simulink model "auvDyn"  (R2018b)
settings: Solver=VariableStepAuto  StartTime=0.0  StopTime=3600  RelTol=1e-3
values from neighbouring files (symbols this model uses):
  aRef = auv.aRef.Value    [auvDyn_ts.m]    (also in hueristicAuvDyn_ts.m)
  AUVmass = auv.AUVmass.Value    [auvDyn_ts.m]    (also in hueristicAuvDyn_ts.m)
  cD = auv.cD.Value    [auvDyn_ts.m]    (also in hueristicAuvDyn_ts.m)
  floorFlow = .5    (= 0.5)    [auvDyn_ts.m]    (also in hueristicAuvDyn_ts.m)
  posOffset = auv.posOffset.Value    [auvDyn_ts.m]    (also in hueristicAuvDyn_ts.m)
  posSP = auv.posSP.Value    [auvDyn_ts.m]    (also in hueristicAuvDyn_ts.m)
  rho = auv.rho.Value    [auvDyn_ts.m]    (also in hueristicAuvDyn_ts.m)
libraries: filteredPIDController_ul x4, vrlib x1, sharedutil x1
settings Model: Creator=jcreed2  LastModifiedBy=jcreed2
settings DataIOCC: SaveOutput=off  DSMLogging=off

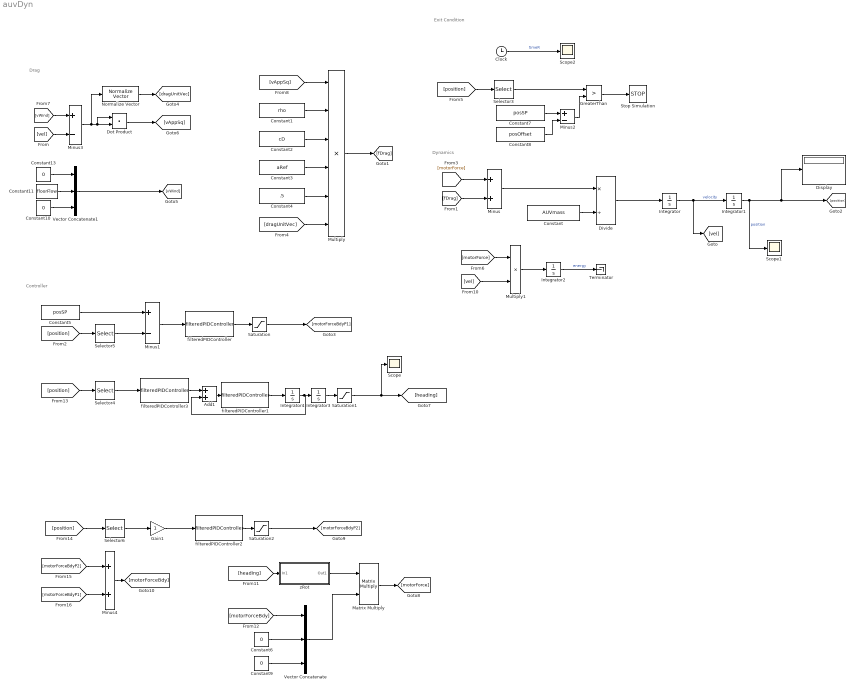
== system auvDyn ==
  note: Exit Condition
  note: Controller
  note: Dynamics
  note: Drag
  Add1 : Sum
  Clock : Clock
  Constant : Constant  Value=AUVmass
  Constant1 : Constant  Value=rho
  Constant{6,9..10,13} (4 alike) : Constant  Value=0
  Constant11 : Constant  Value=floorFlow
  Constant2 : Constant  Value=cD
  Constant3 : Constant  Value=aRef
  Constant4 : Constant  Value=.5
  Constant5 : Constant  Value=posSP
  Constant7 : Constant  Value=posSP
  Constant8 : Constant  Value=posOffset
  Display : Display
  Divide : Product  Inputs=*/
  Dot Product : DotProduct  InputSameDT=on  OutDataTypeStr=Inherit: Inherit via internal rule
  Gain1 : Gain
  GreaterThan : RelationalOperator  Operator=>  OutDataTypeStr=boolean  RndMeth=Simplest
  Integrator{,1..4} (5 alike) : Integrator
  Matrix Multiply : Product  Multiplication=Matrix(*)
  Minus : Sum
  Minus1 : Sum  Inputs=+-
  Minus2 : Sum  Inputs=+-
  Minus3 : Sum  Inputs=+-
  Minus4 : Sum
  Multiply : Product  Inputs=6
  Multiply1 : Product
  Normalize Vector : vrlib/Utilities/Normalize Vector  maxzero=0
      settings: SourceProductName=Simulink 3D Animation  SourceProductBaseCode=VR
  Saturation : Saturate  UpperLimit=7.457*10^3  LowerLimit=0
  Saturation1 : Saturate  UpperLimit=pi/2  LowerLimit=-pi/2
  Saturation2 : Saturate  UpperLimit=7.457*10^3  LowerLimit=0
  Scope : Scope
  Scope1 : Scope
  Scope2 : Scope
  Selector3 : Selector  InputPortWidth=3  IndexOptions=Index vector (dialog)  Indices=[1]  OutputSizes=1
  Selector4 : Selector  InputPortWidth=3  IndexOptions=Index vector (dialog)  Indices=[2]  OutputSizes=1
  Selector5 : Selector  InputPortWidth=3  IndexOptions=Index vector (dialog)  Indices=1  OutputSizes=1
  Selector6 : Selector  InputPortWidth=3  IndexOptions=Index vector (dialog)  Indices=[2]  OutputSizes=1
  Stop Simulation : Stop
  Terminator : Terminator
  Vector Concatenate : Concatenate  NumInputs=3
  Vector Concatenate1 : Concatenate  NumInputs=3
  filteredPIDController : filteredPIDController_ul/filteredPIDController  kp=.8  ki=1*10^-4  kd=3  Value=.001  externalReset=none
  filteredPIDController1 : filteredPIDController_ul/filteredPIDController  kp=.0001  ki=0  kd=0  Value=.001  externalReset=none
  filteredPIDController2 : filteredPIDController_ul/filteredPIDController  kp=6  ki=.01  kd=0  Value=.001  externalReset=none
  filteredPIDController3 : filteredPIDController_ul/filteredPIDController  kp=1e-3  ki=0  kd=5e-6  Value=.001  externalReset=none
  zRot : Subsystem
  wires:
  Integrator/1 -> [vel], Integrator1/1  "velocity"
  Integrator1/1 -> Scope1/1, Display/1, [position]  "position"
  Divide/1 -> Integrator/1
  Constant/1 -> Divide/2
  Minus/1 -> Divide/1
  Constant4/1 -> Multiply/5
  Constant3/1 -> Multiply/4
  Constant2/1 -> Multiply/3
  Constant1/1 -> Multiply/2
  Multiply/1 -> [fDrag]
  [motorForce] -> Minus/1
  [fDrag] -> Minus/2
  Minus1/1 -> filteredPIDController/1
  filteredPIDController/1 -> Saturation/1
  Constant5/1 -> Minus1/1
  Saturation/1 -> [motorForceBdyP1]
  GreaterThan/1 -> Stop Simulation/1
  Constant7/1 -> Minus2/1
  Minus2/1 -> GreaterThan/2
  Constant8/1 -> Minus2/2
  Selector3/1 -> GreaterThan/1
  Clock/1 -> Scope2/1  "timeR"
  [vel] -> Multiply1/2
  Multiply1/1 -> Integrator2/1
  Integrator2/1 -> Terminator/1  "energy"
  [motorForce] -> Multiply1/1
  Minus3/1 -> Dot Product/1, Dot Product/2, Normalize Vector/1
  [vWind] -> Minus3/1
  [vel] -> Minus3/2
  Constant11/1 -> Vector Concatenate1/2
  Constant13/1 -> Vector Concatenate1/1
  Vector Concatenate1/1 -> [vWind]
  Dot Product/1 -> [vAppSq]
  Normalize Vector/1 -> [dragUnitVec]
  [dragUnitVec] -> Multiply/6
  [vAppSq] -> Multiply/1
  Add1/1 -> filteredPIDController1/1
  [heading] -> zRot/1(In1)
  zRot/1(Out1) -> Matrix Multiply/1
  Vector Concatenate/1 -> Matrix Multiply/2
  [motorForceBdy] -> Vector Concatenate/1
  Constant6/1 -> Vector Concatenate/2
  Constant9/1 -> Vector Concatenate/3
  Matrix Multiply/1 -> [motorForce]
  [position] -> Selector3/1
  Constant10/1 -> Vector Concatenate1/3
  Selector5/1 -> Minus1/2
  Selector4/1 -> filteredPIDController3/1
  [position] -> Selector4/1
  [position] -> Selector5/1
  [position] -> Selector6/1
  Selector6/1 -> Gain1/1
  filteredPIDController2/1 -> Saturation2/1
  Saturation2/1 -> [motorForceBdyP2]
  [motorForceBdyP2] -> Minus4/1
  Minus4/1 -> [motorForceBdy]
  [motorForceBdyP1] -> Minus4/2
  Gain1/1 -> filteredPIDController2/1
  Saturation1/1 -> Scope/1, [heading]
  Integrator3/1 -> Saturation1/1
  filteredPIDController3/1 -> Add1/1
  filteredPIDController1/1 -> Integrator4/1
  Integrator4/1 -> Add1/2, Integrator3/1

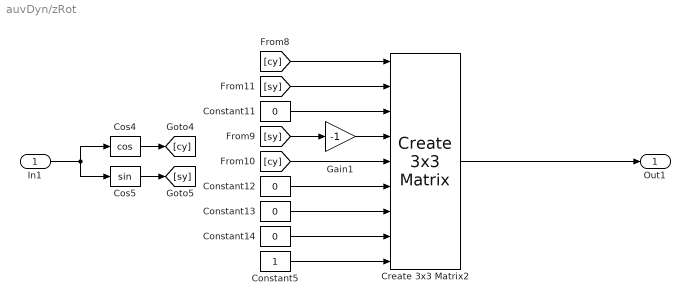
== system auvDyn/zRot ==
  In1 : Inport
  Constant{11..14} (4 alike) : Constant  Value=0
  Constant5 : Constant
  Cos4 : Trigonometry  Operator=cos
  Cos5 : Trigonometry
  Create 3x3 Matrix2 : sharedutil/Create 3x3 Matrix  aMode=aMode
  Gain1 : Gain  Gain=-1
  Out1 : Outport
  wires:
  [cy] -> Create 3x3 Matrix2/5
  [sy] -> Gain1/1
  [sy] -> Create 3x3 Matrix2/2
  Constant12/1 -> Create 3x3 Matrix2/6
  Create 3x3 Matrix2/1 -> Out1/1
  [cy] -> Create 3x3 Matrix2/1
  Constant11/1 -> Create 3x3 Matrix2/3
  Constant14/1 -> Create 3x3 Matrix2/8
  Constant13/1 -> Create 3x3 Matrix2/7
  Gain1/1 -> Create 3x3 Matrix2/4
  Constant5/1 -> Create 3x3 Matrix2/9
  Cos4/1 -> [cy]
  Cos5/1 -> [sy]
  In1/1 -> Cos5/1, Cos4/1
